simulink subsystem "adaptive_flux_wr_observer"  (R2022b)
settings: Solver=VariableStepAuto  StartTime=0.0  StopTime=10.0  RelTol=1e-3
values from neighbouring files (symbols this model uses):
  c = (Lsigma*Lr)/Lm    (= 0.00610975609756)    [im_params_sensorless.m]
  k = 2    [im_params_sensorless.m]
  K1 = (-Rs*Lr^2-Rr*Lm^2)/(Lr*w)    (= -230.46612657)    [im_params_sensorless.m]
  K2 = (Rr*Lm)/(Lr*w)    (= 1155.33638605)    [im_params_sensorless.m]
  K3 = Lm/w    (= 163.672654691)    [im_params_sensorless.m]
  K4 = Lr/w    (= 169.660678643)    [im_params_sensorless.m]
  K5 = Rr*Lm/Lr    (= 0.578823529412)    [im_params_sensorless.m]
  K6 = -Rr/Lr    (= -7.05882352941)    [im_params_sensorless.m]
libraries: slpidlib x1
settings Model: Creator=jack  LastModifiedBy=jack

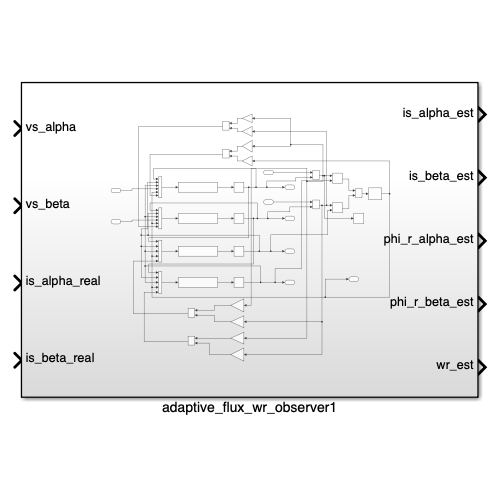
[thumbnail: Simulink's stored preview of the top-level diagram]
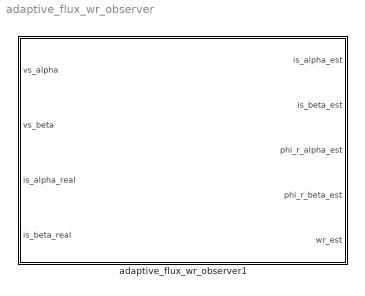
== system adaptive_flux_wr_observer ==
  adaptive_flux_wr_observer1 : Subsystem

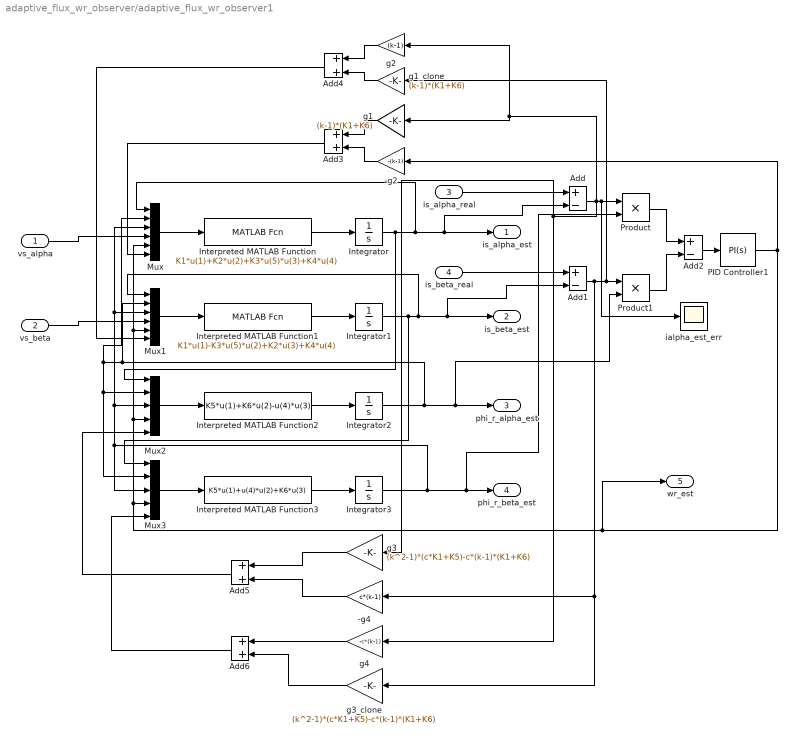
== system adaptive_flux_wr_observer/adaptive_flux_wr_observer1 ==
  vs_alpha : Inport
  vs_beta : Inport  Port=2
  is_alpha_real : Inport  Port=3
  is_beta_real : Inport  Port=4
  -g2 : Gain  Gain=-(k-1)
  -g4 : Gain  Gain=c*(k-1)
  Add : Sum  Inputs=+-
  Add1 : Sum  Inputs=+-
  Add2 : Sum  Inputs=+-
  Add{3..6} (4 alike) : Sum
  Integrator{,1..3} (4 alike) : Integrator
  Interpreted MATLAB Function : MATLABFcn  MATLABFcn=K1*u(1)+K2*u(2)+K3*u(5)*u(3)+K4*u(4)
  Interpreted MATLAB Function1 : MATLABFcn  MATLABFcn=K1*u(1)-K3*u(5)*u(2)+K2*u(3)+K4*u(4)
  Interpreted MATLAB Function2 : MATLABFcn  MATLABFcn=K5*u(1)+K6*u(2)-u(4)*u(3)
  Interpreted MATLAB Function3 : MATLABFcn  MATLABFcn=K5*u(1)+u(4)*u(2)+K6*u(3)
  Mux : Mux  Inputs=6
  Mux1 : Mux  Inputs=6
  Mux2 : Mux  Inputs=5
  Mux3 : Mux  Inputs=5
  PID Controller1 : slpidlib/PID Controller  Controller=PI  Form=Parallel  TimeDomain=Continuous-time  UseExternalTs=off  SampleTime=-1  IntegratorMethod=Forward Euler  FilterMethod=Forward Euler  ControllerParametersSource=internal  P=7*3  I=50*3  UseKiTs=off  D=0  N=100  UseFilter=on  TunerSelectOption=Transfer Function Based (PID Tuner App)  InitialConditionSource=internal  InitialConditionForIntegrator=0  InitialConditionForFilter=0  DifferentiatorICPrevScaledInput=0  ExternalReset=none  TrackingMode=off  Kt=1  LimitOutput=off  SatLimitsSource=internal  UpperSaturationLimit=inf  LowerSaturationLimit=-inf  LinearizeAsGain=on  AntiWindupMode=none  Kb=1  LimitIntegrator=off  UpperIntegratorSaturationLimit=inf  LowerIntegratorSaturationLimit=-inf  POutMin=[]  POutMax=[]  IOutMin=[]  IOutMax=[]  DOutMin=[]  DOutMax=[]  NOutMin=[]  NOutMax=[]  SumOutMin=[]  SumOutMax=[]  SaturationOutMin=[]  SaturationOutMax=[]  PParamMin=[]  PParamMax=[]  IParamMin=[]  IParamMax=[]  DParamMin=[]  DParamMax=[]  NParamMin=[]  NParamMax=[]  KbParamMin=[]  KbParamMax=[]  KtParamMin=[]  KtParamMax=[]  KbOutMin=[]  KbOutMax=[]  KtOutMin=[]  KtOutMax=[]  IntegratorOutMin=[]  IntegratorOutMax=[]  FilterOutMin=[]  FilterOutMax=[]  SumI1OutMin=[]  SumI1OutMax=[]  SumI2OutMin=[]  SumI2OutMax=[]  SumI3OutMin=[]  SumI3OutMax=[]  SumI4OutMin=[]  SumI4OutMax=[]  SumDOutMin=[]  SumDOutMax=[]  DifferentiatorOutMin=[]  DifferentiatorOutMax=[]  FilterDiffOutCoefMin=[]  FilterDiffOutCoefMax=[]  ReciprocalOutMin=[]  ReciprocalOutMax=[]  SumDenOutMin=[]  SumDenOutMax=[]  SumNumOutMin=[]  SumNumOutMax=[]  DivideOutMin=[]  DivideOutMax=[]  UdiffTsProdOutMin=[]  UdiffTsProdOutMax=[]  NTsProdOutMin=[]  NTsProdOutMax=[]  UintegralTsProdOutMin=[]  UintegralTsProdOutMax=[]  UngainTsProdOutMin=[]  UngainTsProdOutMax=[]  ClampingZeroOutDataTypeStr=Inherit: Inherit via back propagation  ClampingZeroOutMin=[]  ClampingZeroOutMax=[]  FilterDenConstantOutDataTypeStr=Inherit: Inherit via back propagation  FilterDenConstantOutMin=[]  FilterDenConstantOutMax=[]  PCopyOutDataTypeStr=Inherit: Inherit via back propagation  PCopyOutMin=[]  PCopyOutMax=[]  NCopyOutDataTypeStr=Inherit: Inherit via back propagation  NCopyOutMin=[]  NCopyOutMax=[]  IntegratorContinuousStateAttributes=''  IntegratorStateMustResolveToSignalObject=off  IntegratorRTWStateStorageClass=Auto  FilterContinuousStateAttributes=''  FilterStateMustResolveToSignalObject=off  FilterRTWStateStorageClass=Auto  ParallelPVariant=InternalParameters  IdealPVariant=Disabled  IVariant=InternalParameters  DVariant=Disabled  IntegratorVariant=Continuous  SatVariant=Disabled  AWVariant=Passthrough  PCopyVariant=Disabled  TRVariant=Disabled  FdbkBlocksVariant=Forward  IdealPFdbkVariant=Disabled  SatFdbkVariant=Disabled  DerivativeFilterVariant=Disabled  NVariant=Disabled  NCopyVariant=Disabled_SignalSpec  FilterICVariant=Disabled  IntegratorICVariant=InternalICs  ExternalResetVariant=Disabled  TRSumVariant=Passthrough  SumFdbkVariant=Disabled  SumVariant=Sum_PI  TsampFilterVariant=InternalTs  TsampNgainVariant=Passthrough  TsampIntegralVariant=Passthrough  ExternalSaturationOutDataTypeStr=Inherit: Same as second input
  Product : Product
  Product1 : Product
  g1 : Gain  Gain=(k-1)*(K1+K6)
  g1_clone : Gain  Gain=(k-1)*(K1+K6)
  g2 : Gain  Gain=(k-1)
  g3 : Gain  Gain=(k^2-1)*(c*K1+K5)-c*(k-1)*(K1+K6)
  g3_clone : Gain  Gain=(k^2-1)*(c*K1+K5)-c*(k-1)*(K1+K6)
  g4 : Gain  Gain=-c*(k-1)
  ialpha_est_err : Scope
  is_alpha_est : Outport
  is_beta_est : Outport  Port=2
  phi_r_alpha_est : Outport  Port=3
  phi_r_beta_est : Outport  Port=4
  wr_est : Outport  Port=5
  wires:
  Add3/1 -> Mux/6
  is_alpha_real/1 -> Add/1
  Mux1/1 -> Interpreted MATLAB Function1/1
  Interpreted MATLAB Function1/1 -> Integrator1/1
  Mux/1 -> Interpreted MATLAB Function/1
  Product1/1 -> Add2/2
  Integrator3/1 -> phi_r_beta_est/1, Product/2, Mux3/3, Mux2/3, Mux/3, Mux1/3
  vs_beta/1 -> Mux1/4
  Add5/1 -> Mux2/5
  Add/1 -> g3/1, g4/1, g2/1, g1/1, ialpha_est_err/1, Product/1
  is_beta_real/1 -> Add1/1
  Add4/1 -> Mux1/6
  g3/1 -> Add5/1
  g1_clone/1 -> Add4/2
  Integrator/1 -> Mux2/1, is_alpha_est/1, Add/2, Mux/1
  g1/1 -> Add3/1
  Interpreted MATLAB Function3/1 -> Integrator3/1
  g4/1 -> Add6/1
  Interpreted MATLAB Function/1 -> Integrator/1
  vs_alpha/1 -> Mux/4
  Add2/1 -> PID Controller1/1
  PID Controller1/1 -> wr_est/1, Mux3/4, Mux2/4, Mux1/5, Mux/5, -g2/1
  -g4/1 -> Add5/2
  Mux3/1 -> Interpreted MATLAB Function3/1
  g2/1 -> Add4/1
  Add6/1 -> Mux3/5
  Interpreted MATLAB Function2/1 -> Integrator2/1
  Integrator2/1 -> phi_r_alpha_est/1, Product1/2, Mux1/2, Mux/2, Mux3/2, Mux2/2
  Mux2/1 -> Interpreted MATLAB Function2/1
  -g2/1 -> Add3/2
  Product/1 -> Add2/1
  Integrator1/1 -> Mux3/1, is_beta_est/1, Add1/2, Mux1/1
  Add1/1 -> -g4/1, g3_clone/1, g1_clone/1, Product1/1
  g3_clone/1 -> Add6/2
